simulink model "sampleModel1727_2_sub_sub_sub"  (R2023a)
settings: Solver=VariableStepAuto  StartTime=0.0  StopTime=10.0  RelTol=1e-3
libraries: simulink x4, hdlsllib x3
settings Model: Creator=user1  LastModifiedBy=user1

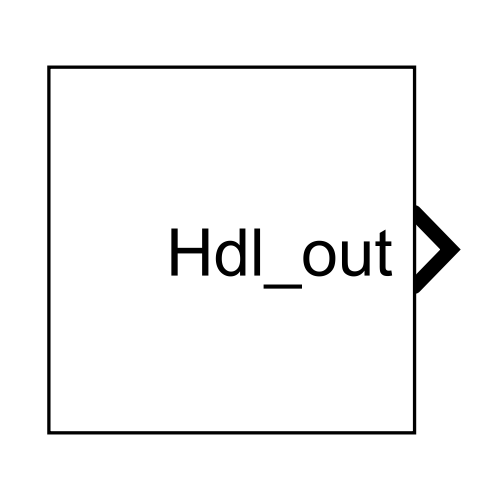
[thumbnail: Simulink's stored preview of the top-level diagram]
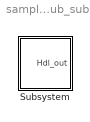
== system sampleModel1727_2_sub_sub_sub ==
  Subsystem : Subsystem

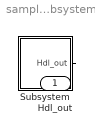
== system sampleModel1727_2_sub_sub_sub/Subsystem ==
  Subsystem : Subsystem
  Hdl_out : Outport  OutDataTypeStr=uint8
  wires:
  Subsystem/1(Hdl_out) -> Hdl_out/1

== system sampleModel1727_2_sub_sub_sub/Subsystem/Subsystem ==
  Subsystem : Subsystem
  Hdl_out : Outport  OutDataTypeStr=uint8

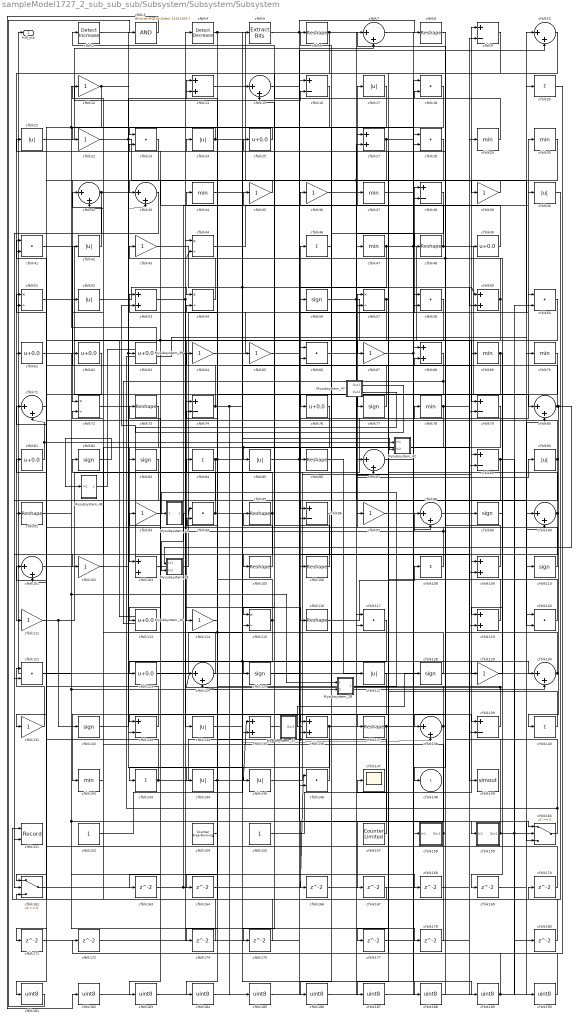
== system sampleModel1727_2_sub_sub_sub/Subsystem/Subsystem/Subsystem ==
  Mysubsystem_10 : Subsystem  TreatAsAtomicUnit=on  RTWFcnName=Mysubsystem_10
      settings: RTWFcnNameOpts=User specified  RTWFileNameOpts=Use function name
  Mysubsystem_11 : Subsystem  TreatAsAtomicUnit=on  RTWFcnName=Mysubsystem_11
      settings: RTWFcnNameOpts=User specified  RTWFileNameOpts=Use function name
  Mysubsystem_28 : Subsystem  TreatAsAtomicUnit=on  RTWFcnName=Mysubsystem_28
      settings: RTWFcnNameOpts=User specified  RTWFileNameOpts=Use function name
  Mysubsystem_31 : Subsystem  TreatAsAtomicUnit=on  RTWFcnName=Mysubsystem_31
      settings: RTWFcnNameOpts=User specified  RTWFileNameOpts=Use function name
  Mysubsystem_38 : Subsystem  TreatAsAtomicUnit=on  RTWFcnName=Mysubsystem_38
      settings: RTWFcnNameOpts=User specified  RTWFileNameOpts=Use function name
  Mysubsystem_39 : Subsystem  TreatAsAtomicUnit=on  RTWFcnName=Mysubsystem_39
      settings: RTWFcnNameOpts=User specified  RTWFileNameOpts=Use function name
  Mysubsystem_40 : Subsystem  TreatAsAtomicUnit=on  RTWFcnName=Mysubsystem_40
      settings: RTWFcnNameOpts=User specified  RTWFileNameOpts=Use function name
  Mysubsystem_42 : Subsystem  TreatAsAtomicUnit=on  RTWFcnName=Mysubsystem_42
      settings: RTWFcnNameOpts=User specified  RTWFileNameOpts=Use function name
  Mysubsystem_47 : Subsystem  TreatAsAtomicUnit=on  RTWFcnName=Mysubsystem_47
      settings: RTWFcnNameOpts=User specified  RTWFileNameOpts=Use function name
  cfblk{7,10,15,32..33,71,80,87,98,100..101,124,130,138} (14 alike) : Sum  Inputs=|++  OutDataTypeStr=uint8
  cfblk{12,22,35..36,39,43,64..65,67,93,97,102,111,114,129,131} (16 alike) : Gain  OutDataTypeStr=uint8
  cfblk{14,27,53,59,68,103,109,119,135..136} (10 alike) : Sum  OutDataTypeStr=uint8
  cfblk{6,8,48,73,86,91,95,105..106,116,137} (11 alike) : Reshape
  cfblk{20,46,84,108,140,143} (6 alike) : Sum  Inputs=+  OutDataTypeStr=uint8
  cfblk{56,77,82..83,99,110,125,128,132} (9 alike) : Signum
  cfblk{25,49,61..63,76,81,113,123} (9 alike) : Bias  Bias=0.0  SaturateOnIntegerOverflow=off
  cfblk{44,51,54,57,72,115} (6 alike) : Product  Inputs=*/  OutDataTypeStr=uint8  RndMeth=Zero  SaturateOnIntegerOverflow=on
  cfblk{18,23,28,41,58,60,66,94,117,120..121,146} (12 alike) : DotProduct  OutDataTypeStr=uint8
  cfblk{17,21,24,40,42,52,85,90,127,134,144..145} (12 alike) : Abs  OutDataTypeStr=uint8  SaturateOnIntegerOverflow=off
  cfblk{9,16,38,74,79,89,96,133,139} (9 alike) : Sum  Inputs=+-  OutDataTypeStr=uint8
  cfblk{29..30,34,37,47,69..70,78,142} (9 alike) : MinMax  OutDataTypeStr=uint8
  cfblk147 : Scope
  cfblk149 : ToWorkspace  VariableName=simout  SaveFormat=Timeseries  SampleTime=-1
  cfblk151 : Record  FileSettingsInternal="{\"entries\":[{\"content\":{\"excelSettings\":{\"content\":{},\"type\":\"Streamout.ExcelSettings\"}},\"type\":\"Streamout.FileSettingStorage\",\"uuid\":\"\"}],\"packageUris\":[\"http:\\/\\/schema.mathworks.com\\/mf0\\/streamout_blocks\\/R2020a\"],\"version\":\"1.0\"}"  Layout=[1 1]  SignalsInternal="{\"entries\":[{\"content\":{\"signals\":[{\"content\":{\"blockPath\":[],\"dimensions\":[1],\"domain\":\"\",\"lineColor\":\"#a2142f\",\"plots\":[1],\"port\":1,\"signalID\":37443,\"signalName\":\"cfblk158\"},\"type\":\"RecordBlkView.Signal\",\"uuid\":\"\"},{\"content\":{\"blockPath\":[],\"dimensions\":[1],\"domain\":\"\",\"lineColor\":\"#139fff\",\"plots\":[1],\"port\":2,\"signalID\":37446,\"signalName\":\"cfblk100\"},\"type\":\"RecordBlkView.Signal\",\"uuid\":\"\"}]},\"type\":\"RecordBlkView.InputSignals\",\"uuid\":\"\"}],\"packageUris\":[\"http:\\/\\/schema.mathworks.com\\/mf0\\/streamout_blocks\\/R2020a\"],\"version\":\"1.0\"}"  VisualizationBindings="{\"xyplotplugin\":{\"info\":[{\"series\":[{\"bindingParametersList\":[{\"parameter\":\"X-Axis\",\"signalID\":37443,\"signalName\":\"cfblk158\"},{\"parameter\":\"Y-Axis\",\"signalID\":37446,\"signalName\":\"cfblk100\"}],\"seriesID\":422}],\"subplotID\":1}]}}"  CompatibilityTag=XY  st=-1
  cfblk152 : Constant  OutDataTypeStr=uint8  SampleTime=-1
  cfblk154 : hdlsllib/Sources/Counter Free-Running  NumBits=16  tsamp=-1
  cfblk155 : Constant  OutDataTypeStr=uint8  SampleTime=-1
  cfblk157 : hdlsllib/Sources/Counter Limited  uplimit=7  tsamp=-1
  cfblk158 : Subsystem
      settings: LibrarySourceBlock=|
      | hdlsllib/Ports &
      | Subsystems/Subsystem
  cfblk159 : Subsystem
      settings: LibrarySourceBlock=|
      | hdlsllib/Ports &
      | Subsystems/Subsystem
  cfblk160 : Switch  OutDataTypeStr=uint8  SaturateOnIntegerOverflow=off  InputSameDT=off
  cfblk161 : Switch  OutDataTypeStr=uint8  SaturateOnIntegerOverflow=off  InputSameDT=off
  cfblk{163..164,166..172,174..175,177..178,180} (14 alike) : Delay  SampleTime=1
  cfblk{181..190} (10 alike) : DataTypeConversion  OutDataTypeStr=uint8  SaturateOnIntegerOverflow=off  RndMeth=Floor
  cfblk2 : simulink/Logic and Bit Operations/Detect Increase  vinit=0.0  OutDataTypeStr=uint8
      settings: LibrarySourceBlock=|
      | hdlsllib/Logic and Bit
      | Operations/Detect
      | Increase
  cfblk3 : simulink/Logic and Bit Operations/Bitwise Operator  logicop=AND  UseBitMask=on  BitMask=bin2dec('11011001')  BitMaskRealWorld=Stored Integer
      settings: LibrarySourceBlock=|
      | hdlsllib/Logic and Bit
      | Operations/Bitwise
      | Operator
  cfblk4 : simulink/Logic and Bit Operations/Detect Decrease  vinit=0.0  OutDataTypeStr=uint8
      settings: LibrarySourceBlock=|
      | hdlsllib/Logic and Bit
      | Operations/Detect
      | Decrease
  cfblk5 : simulink/Logic and Bit Operations/Extract Bits  bitsToExtract=Upper half  numBits=8  bitIdxRange=[0 7]  outScalingMode=Preserve fixed-point scaling
      settings: LibrarySourceBlock=|
      | hdlsllib/Logic and Bit
      | Operations/Extract Bits
  cfblk148 : Outport  OutDataTypeStr=uint8  VectorParamsAs1DForOutWhenUnconnected=off
  Hdl_out : Outport  Port=2  OutDataTypeStr=uint8
  wires:
  cfblk108/1 -> cfblk94/1, cfblk57/1
  cfblk161/1 -> cfblk146/1, cfblk35/1
  cfblk155/1 -> cfblk9/1
  cfblk52/1 -> cfblk54/1
  cfblk6/1 -> cfblk111/1, cfblk38/2, cfblk59/2
  cfblk73/1 -> cfblk103/1
  cfblk86/1 -> cfblk127/1
  cfblk69/1 -> cfblk119/1, cfblk148/1
  cfblk35/1 -> cfblk72/1
  cfblk49/1 -> cfblk17/1
  cfblk57/1 -> cfblk177/1, cfblk114/1
  cfblk120/1 -> cfblk109/1
  cfblk39/1 -> cfblk33/1
  cfblk42/1 -> cfblk32/1
  cfblk79/1 -> cfblk85/1, cfblk113/1
  cfblk10/1 -> cfblk137/1
  cfblk95/1 -> cfblk115/2, cfblk82/1
  cfblk41/1 -> cfblk77/1
  cfblk27/1 -> cfblk146/2, cfblk158/1(In1)
  cfblk74/1 -> cfblk42/1, cfblk185/1, cfblk159/1(In1)
  cfblk111/1 -> cfblk132/1, cfblk30/1
  cfblk29/1 -> cfblk2/1
  cfblk116/1 -> cfblk108/1
  cfblk103/1 -> cfblk60/1
  cfblk139/1 -> cfblk124/1, cfblk53/1
  cfblk4/1 -> cfblk124/2, cfblk39/1
  cfblk9/1 -> cfblk105/1
  cfblk33/1 -> cfblk61/1
  cfblk132/1 -> cfblk14/2, cfblk63/1
  cfblk71/1 -> cfblk161/1
  cfblk143/1 -> cfblk5/1, cfblk101/1
  cfblk146/1 -> cfblk74/2, cfblk46/1
  cfblk105/1 -> cfblk95/1
  cfblk77/1 -> cfblk6/1
  cfblk110/1 -> cfblk51/1
  cfblk51/1 -> cfblk67/1
  cfblk37/1 -> cfblk189/1
  cfblk64/1 -> cfblk20/1
  cfblk121/1 -> cfblk178/1, cfblk160/2, Mysubsystem_28/2(In2)
  cfblk154/1 -> cfblk34/1
  cfblk59/1 -> cfblk15/2, cfblk131/1
  cfblk159/1(Out1) -> cfblk97/1, cfblk180/1, cfblk80/2
  cfblk23/1 -> cfblk101/2
  cfblk78/1 -> cfblk102/1, cfblk149/1
  cfblk80/1 -> cfblk41/1, cfblk140/1, Mysubsystem_38/1(In1)
  cfblk68/1 -> cfblk144/1, Mysubsystem_10/2(In2)
  cfblk14/1 -> cfblk70/1
  cfblk43/1 -> cfblk98/2
  cfblk28/1 -> cfblk123/1
  cfblk158/1(Out1) -> cfblk52/1, cfblk151/1
  cfblk38/1 -> cfblk76/1
  cfblk60/1 -> cfblk133/1, Mysubsystem_10/1(In1)
  cfblk56/1 -> cfblk80/1, cfblk79/1
  cfblk48/1 -> cfblk23/2, cfblk120/1
  cfblk123/1 -> cfblk15/1
  cfblk152/1 -> cfblk65/1
  cfblk144/1 -> cfblk64/1, cfblk135/1
  cfblk97/1 -> cfblk68/1
  cfblk142/1 -> cfblk32/2
  cfblk157/1 -> cfblk84/1
  cfblk113/1 -> cfblk93/1
  cfblk12/1 -> cfblk145/1, cfblk91/1
  cfblk100/1 -> cfblk56/1, cfblk151/2
  cfblk46/1 -> cfblk86/1
  cfblk133/1 -> cfblk81/1
  cfblk160/1 -> cfblk21/1, Mysubsystem_39/2(In2)
  cfblk125/1 -> cfblk89/1
  cfblk63/1 -> cfblk38/1
  cfblk47/1 -> cfblk96/2, cfblk40/1, cfblk99/1
  cfblk34/1 -> cfblk89/2
  cfblk84/1 -> cfblk133/2, cfblk188/1, cfblk184/1
  cfblk115/1 -> cfblk94/2, cfblk174/1, cfblk135/2
  cfblk135/1 -> cfblk47/1
  cfblk66/1 -> cfblk100/2
  cfblk119/1 -> cfblk27/1
  cfblk32/1 -> cfblk121/2, cfblk130/1
  cfblk145/1 -> cfblk57/2
  cfblk101/1 -> cfblk160/3, Mysubsystem_28/1(In1)
  cfblk87/1 -> cfblk58/1
  cfblk128/1 -> cfblk24/1, cfblk73/1
  cfblk138/1 -> cfblk166/1, cfblk36/1
  cfblk90/1 -> cfblk41/2, cfblk143/1
  cfblk83/1 -> cfblk161/2
  cfblk94/1 -> cfblk62/1, Mysubsystem_42/2(In2)
  cfblk7/1 -> cfblk58/2
  cfblk54/1 -> cfblk43/1
  cfblk93/1 -> cfblk134/1
  cfblk76/1 -> cfblk115/1
  cfblk15/1 -> cfblk160/1
  cfblk114/1 -> cfblk14/1
  cfblk131/1 -> cfblk121/1
  cfblk44/1 -> cfblk10/1
  cfblk109/1 -> cfblk44/2, cfblk7/1
  cfblk22/1 -> cfblk87/2, cfblk33/2
  cfblk21/1 -> cfblk7/2
  cfblk2/1 -> cfblk125/1
  cfblk134/1 -> cfblk69/1
  cfblk129/1 -> cfblk49/1
  cfblk67/1 -> cfblk129/1, cfblk28/1
  cfblk85/1 -> cfblk139/1, cfblk78/1
  cfblk130/1 -> Hdl_out/1, cfblk68/2
  cfblk102/1 -> cfblk83/1
  cfblk25/1 -> cfblk22/1
  cfblk136/1 -> cfblk163/1, cfblk90/1
  cfblk106/1 -> cfblk25/1
  cfblk89/1 -> cfblk190/1, cfblk136/2
  cfblk24/1 -> cfblk23/1, cfblk138/2, cfblk59/1
  cfblk137/1 -> cfblk167/1, cfblk139/2
  cfblk91/1 -> cfblk130/2
  cfblk5/1 -> cfblk109/2, cfblk8/1
  cfblk30/1 -> cfblk96/1
  cfblk53/1 -> cfblk116/1, cfblk4/1
  cfblk72/1 -> cfblk136/1
  cfblk16/1 -> cfblk66/2
  cfblk127/1 -> cfblk142/1
  cfblk8/1 -> cfblk138/1
  cfblk81/1 -> cfblk71/2, Mysubsystem_42/1(In1)
  cfblk98/1 -> cfblk29/1
  cfblk140/1 -> cfblk87/1
  cfblk65/1 -> cfblk10/2
  cfblk36/1 -> cfblk48/1
  cfblk124/1 -> cfblk12/1
  cfblk163/1 -> cfblk66/1
  cfblk58/1 -> cfblk164/1
  cfblk164/1 -> cfblk27/2
  cfblk166/1 -> cfblk79/2
  cfblk167/1 -> cfblk161/3
  cfblk61/1 -> cfblk168/1
  cfblk168/1 -> cfblk98/1
  cfblk99/1 -> cfblk169/1
  cfblk169/1 -> cfblk100/1
  cfblk40/1 -> cfblk170/1
  cfblk170/1 -> cfblk71/1
  cfblk96/1 -> cfblk171/1
  cfblk171/1 -> cfblk44/1
  cfblk20/1 -> cfblk172/1
  cfblk172/1 -> cfblk16/1
  cfblk174/1 -> cfblk72/2
  cfblk17/1 -> cfblk175/1
  cfblk175/1 -> cfblk51/2
  cfblk177/1 -> cfblk119/2
  cfblk178/1 -> cfblk54/2
  cfblk180/1 -> cfblk74/1
  cfblk62/1 -> cfblk181/1
  cfblk181/1 -> cfblk3/1
  cfblk3/1 -> cfblk182/1
  cfblk182/1 -> cfblk110/1
  cfblk117/1 -> cfblk183/1
  cfblk183/1 -> cfblk106/1
  cfblk184/1 -> cfblk117/1
  cfblk185/1 -> cfblk117/2
  cfblk18/1 -> cfblk186/1
  cfblk186/1 -> cfblk9/2
  cfblk70/1 -> cfblk187/1
  cfblk187/1 -> cfblk18/1
  cfblk188/1 -> cfblk18/2
  cfblk189/1 -> cfblk60/2, cfblk147/1
  cfblk190/1 -> cfblk37/1
  Mysubsystem_28/1(Out1) -> Mysubsystem_11/1(In1)
  Mysubsystem_31/1(Out1) -> cfblk128/1
  Mysubsystem_11/1(Out1) -> Mysubsystem_38/2(In2)
  Mysubsystem_39/1(Out1) -> cfblk28/2, cfblk16/2
  Mysubsystem_39/2(Out2) -> cfblk120/2
  cfblk82/1 -> Mysubsystem_40/1(In1)
  Mysubsystem_40/1(y) -> Mysubsystem_39/1(In1)
  Mysubsystem_47/1(Out1) -> cfblk53/2
  Mysubsystem_47/2(Out2) -> cfblk103/2

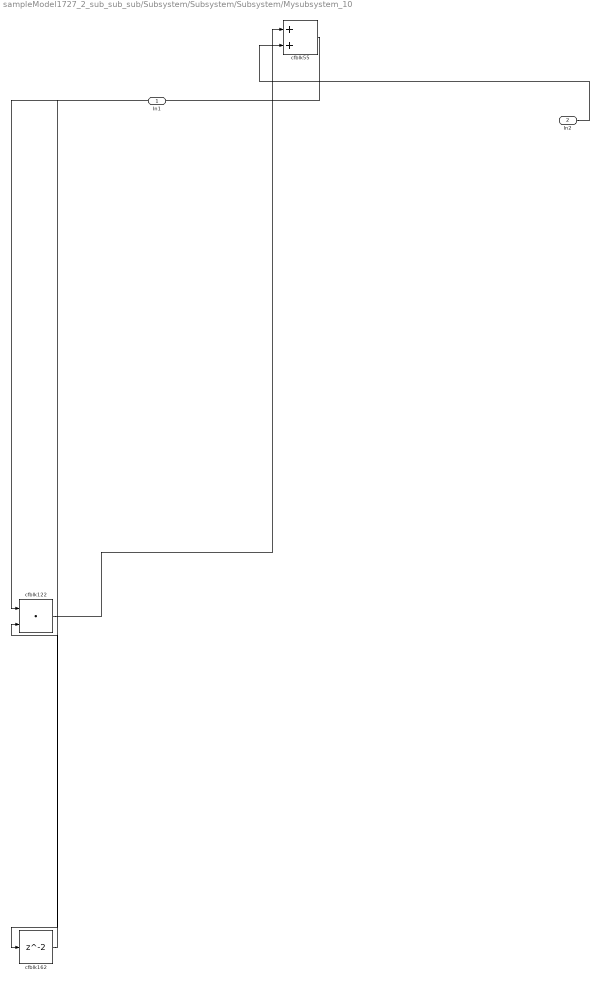
== system sampleModel1727_2_sub_sub_sub/Subsystem/Subsystem/Subsystem/Mysubsystem_10 ==
  In1 : Inport
  In2 : Inport  Port=2
  cfblk122 : DotProduct  OutDataTypeStr=Inherit: Inherit via internal rule
  cfblk162 : Delay  SampleTime=1
  cfblk55 : Sum
  wires:
  In2/1 -> cfblk55/2
  In1/1 -> cfblk122/1
  cfblk162/1 -> cfblk122/2
  cfblk122/1 -> cfblk55/1
  cfblk55/1 -> cfblk162/1

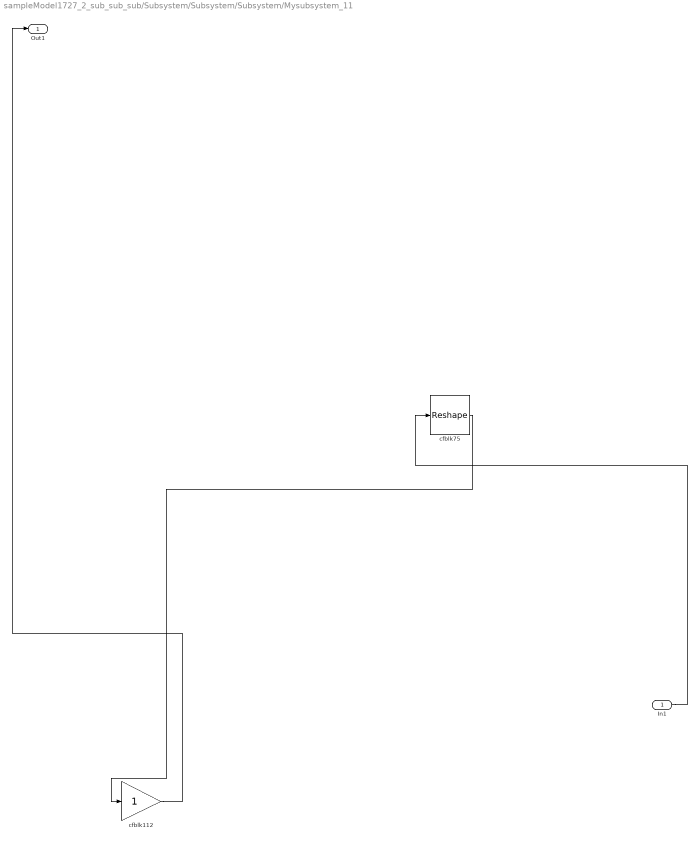
== system sampleModel1727_2_sub_sub_sub/Subsystem/Subsystem/Subsystem/Mysubsystem_11 ==
  In1 : Inport
  cfblk112 : Gain
  cfblk75 : Reshape
  Out1 : Outport
  wires:
  In1/1 -> cfblk75/1
  cfblk112/1 -> Out1/1
  cfblk75/1 -> cfblk112/1

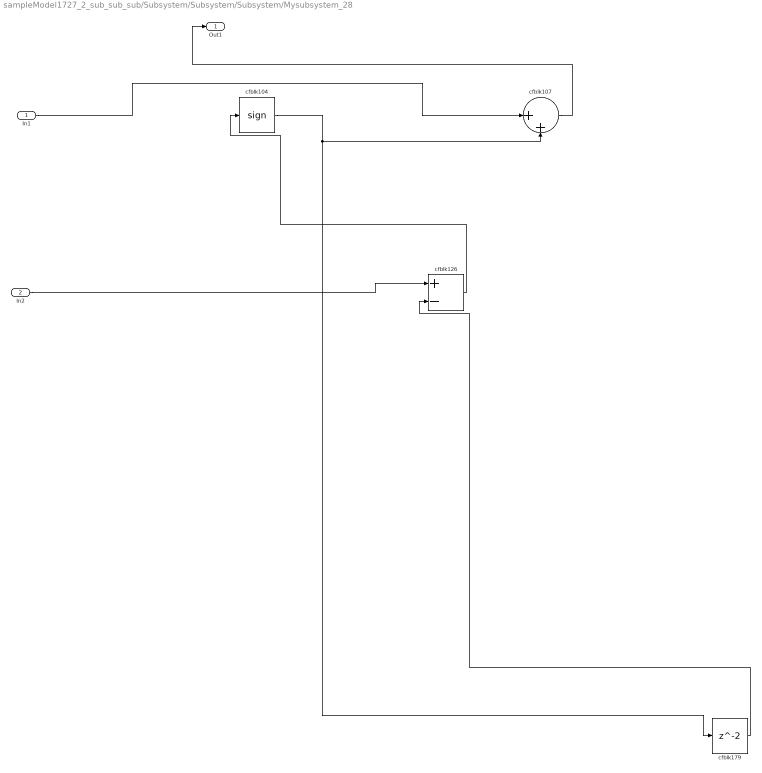
== system sampleModel1727_2_sub_sub_sub/Subsystem/Subsystem/Subsystem/Mysubsystem_28 ==
  In1 : Inport
  In2 : Inport  Port=2
  cfblk104 : Signum
  cfblk107 : Sum  Inputs=|++
  cfblk126 : Sum  Inputs=+-
  cfblk179 : Delay  SampleTime=1
  Out1 : Outport
  wires:
  cfblk104/1 -> cfblk179/1, cfblk107/2
  In2/1 -> cfblk126/1
  In1/1 -> cfblk107/1
  cfblk107/1 -> Out1/1
  cfblk126/1 -> cfblk104/1
  cfblk179/1 -> cfblk126/2

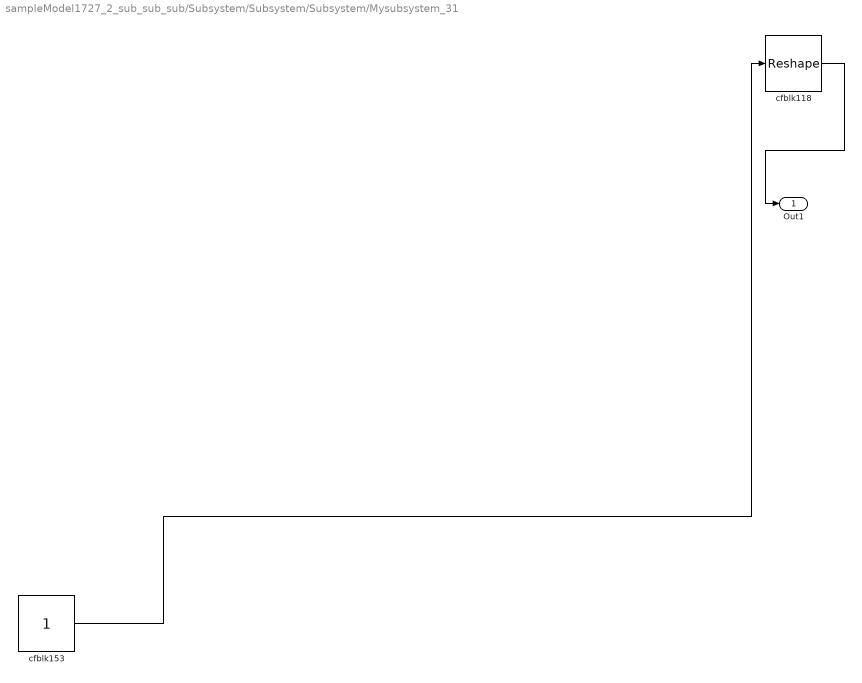
== system sampleModel1727_2_sub_sub_sub/Subsystem/Subsystem/Subsystem/Mysubsystem_31 ==
  cfblk118 : Reshape
  cfblk153 : Constant  SampleTime=-1
  Out1 : Outport
  wires:
  cfblk118/1 -> Out1/1
  cfblk153/1 -> cfblk118/1

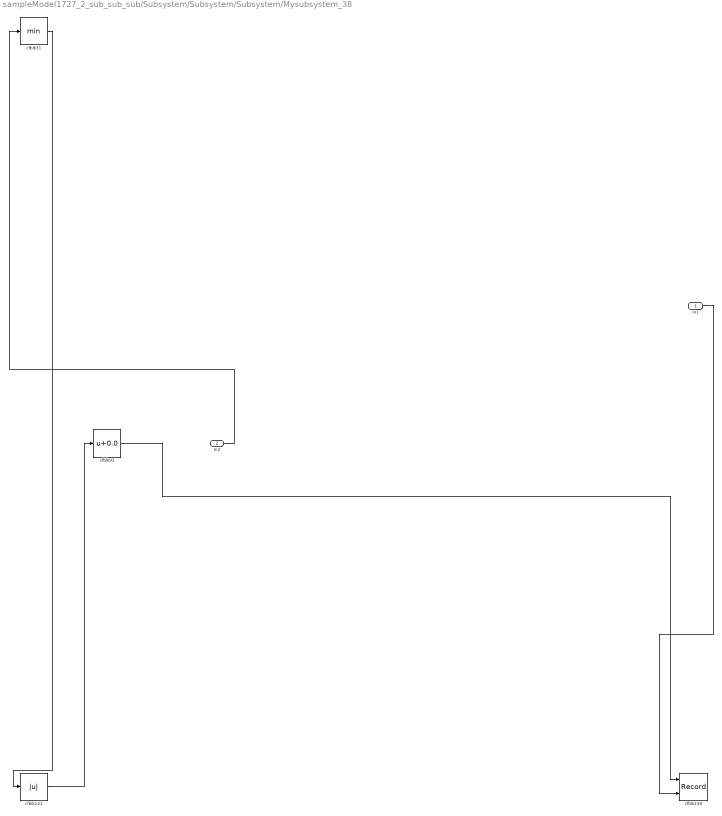
== system sampleModel1727_2_sub_sub_sub/Subsystem/Subsystem/Subsystem/Mysubsystem_38 ==
  In1 : Inport
  In2 : Inport  Port=2
  cfblk141 : Abs  SaturateOnIntegerOverflow=off
  cfblk150 : Record  FileSettingsInternal="{\"entries\":[{\"content\":{\"excelSettings\":{\"content\":{},\"type\":\"Streamout.ExcelSettings\"}},\"type\":\"Streamout.FileSettingStorage\",\"uuid\":\"\"}],\"packageUris\":[\"http:\\/\\/schema.mathworks.com\\/mf0\\/streamout_blocks\\/R2020a\"],\"version\":\"1.0\"}"  Layout=[1 1]  SignalsInternal="{\"entries\":[{\"content\":{},\"type\":\"RecordBlkView.InputSignals\",\"uuid\":\"\"}],\"packageUris\":[\"http:\\/\\/schema.mathworks.com\\/mf0\\/streamout_blocks\\/R2020a\"],\"version\":\"1.0\"}"  VisualizationBindings="{\"xyplotplugin\":{\"info\":[{\"series\":[],\"subplotID\":1}]}}"  CompatibilityTag=XY  st=-1
  cfblk31 : MinMax
  cfblk92 : Bias  Bias=0.0  SaturateOnIntegerOverflow=off
  wires:
  In1/1 -> cfblk150/2
  In2/1 -> cfblk31/1
  cfblk31/1 -> cfblk141/1
  cfblk92/1 -> cfblk150/1
  cfblk141/1 -> cfblk92/1

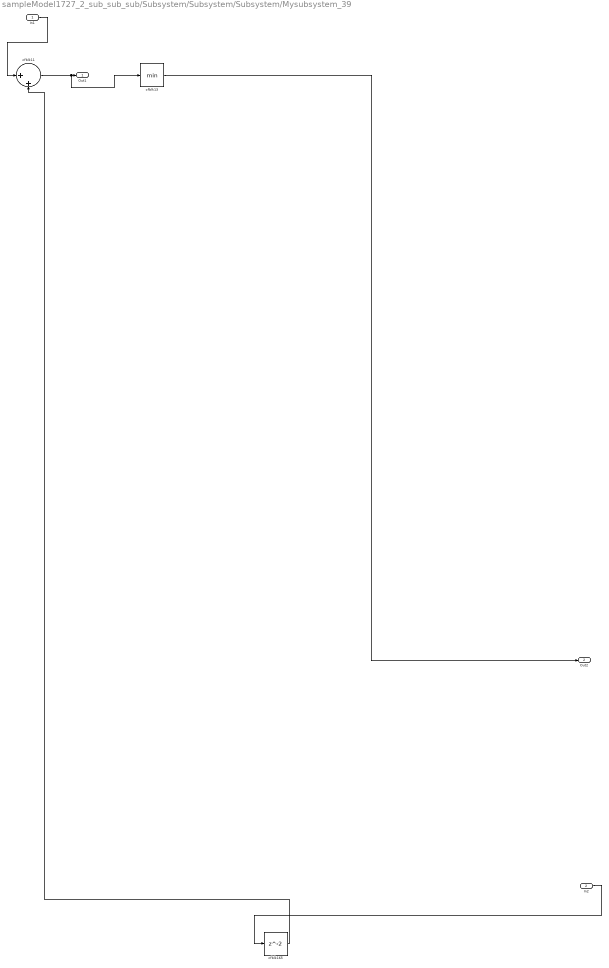
== system sampleModel1727_2_sub_sub_sub/Subsystem/Subsystem/Subsystem/Mysubsystem_39 ==
  In1 : Inport
  In2 : Inport  Port=2
  cfblk11 : Sum  Inputs=|++
  cfblk13 : MinMax
  cfblk165 : Delay  SampleTime=1
  Out1 : Outport
  Out2 : Outport  Port=2
  wires:
  cfblk11/1 -> Out1/1, cfblk13/1
  In2/1 -> cfblk165/1
  cfblk13/1 -> Out2/1
  cfblk165/1 -> cfblk11/2
  In1/1 -> cfblk11/1

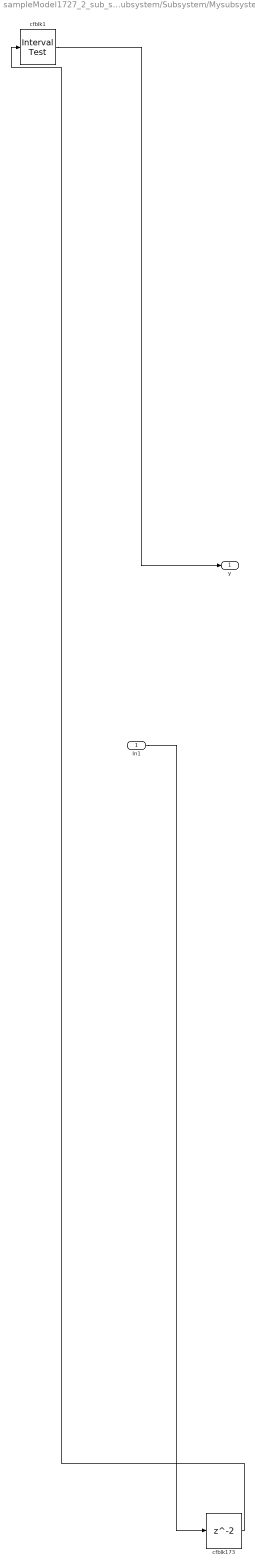
== system sampleModel1727_2_sub_sub_sub/Subsystem/Subsystem/Subsystem/Mysubsystem_40 ==
  In1 : Inport
  cfblk1 : hdlsllib/Logic and Bit Operations/Interval Test  IntervalClosedRight=on  uplimit=0.5  IntervalClosedLeft=on  lowlimit=-0.5  OutDataTypeStr=boolean
  cfblk173 : Delay  SampleTime=1
  y : Outport
  wires:
  In1/1 -> cfblk173/1
  cfblk1/1 -> y/1
  cfblk173/1 -> cfblk1/1

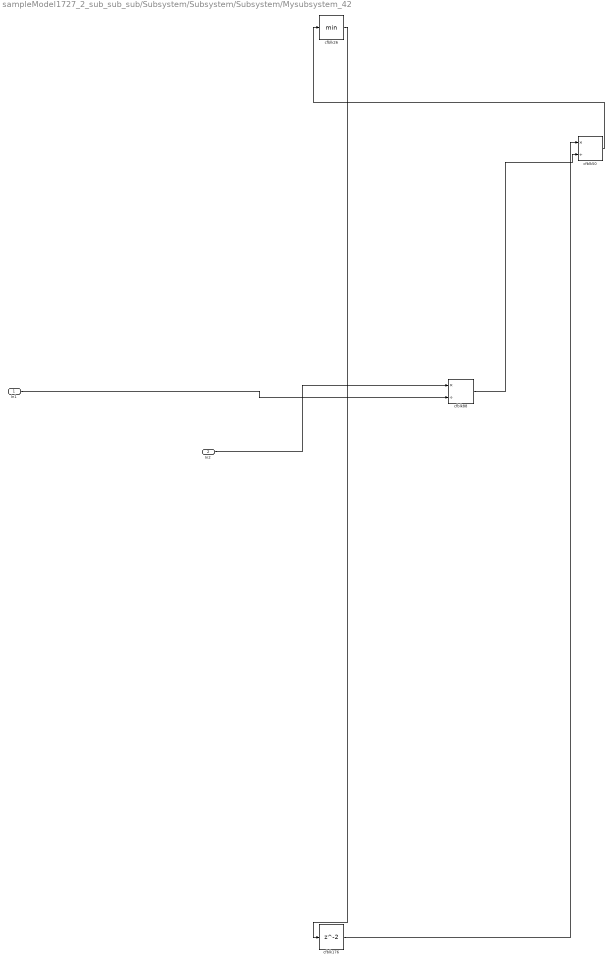
== system sampleModel1727_2_sub_sub_sub/Subsystem/Subsystem/Subsystem/Mysubsystem_42 ==
  In1 : Inport
  In2 : Inport  Port=2
  cfblk176 : Delay  SampleTime=1
  cfblk26 : MinMax
  cfblk50 : Product  Inputs=*/  RndMeth=Zero  SaturateOnIntegerOverflow=on
  cfblk88 : Product  Inputs=*/  RndMeth=Zero  SaturateOnIntegerOverflow=on
  wires:
  In1/1 -> cfblk88/2
  cfblk50/1 -> cfblk26/1
  cfblk88/1 -> cfblk50/2
  In2/1 -> cfblk88/1
  cfblk26/1 -> cfblk176/1
  cfblk176/1 -> cfblk50/1

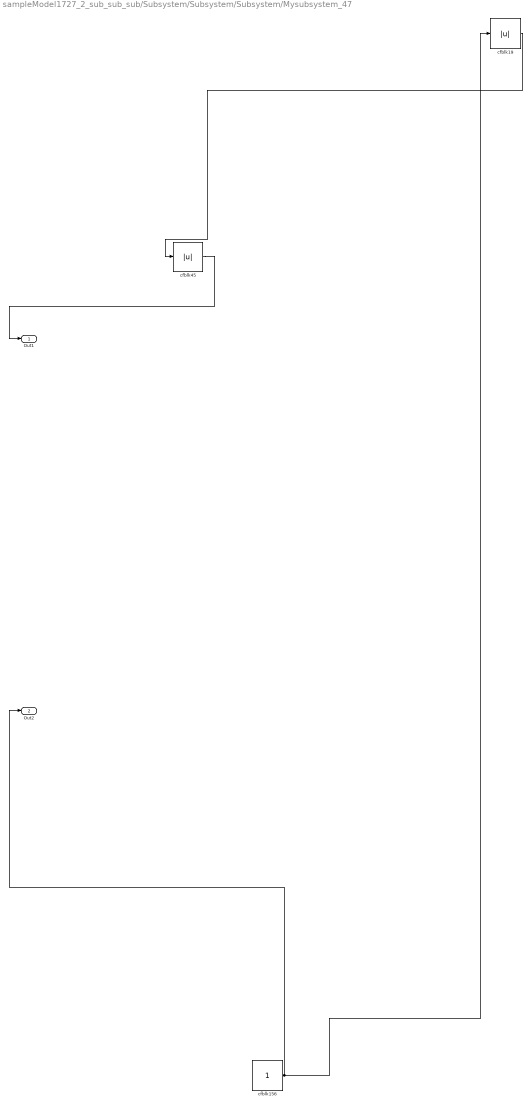
== system sampleModel1727_2_sub_sub_sub/Subsystem/Subsystem/Subsystem/Mysubsystem_47 ==
  cfblk156 : Constant  SampleTime=-1
  cfblk19 : Abs  SaturateOnIntegerOverflow=off
  cfblk45 : Abs  SaturateOnIntegerOverflow=off
  Out1 : Outport
  Out2 : Outport  Port=2
  wires:
  cfblk156/1 -> cfblk19/1, Out2/1
  cfblk19/1 -> cfblk45/1
  cfblk45/1 -> Out1/1

== system sampleModel1727_2_sub_sub_sub/Subsystem/Subsystem/Subsystem/cfblk158 ==
  In1 : Inport
  Out1 : Outport
  wires:
  In1/1 -> Out1/1

== system sampleModel1727_2_sub_sub_sub/Subsystem/Subsystem/Subsystem/cfblk159 ==
  In1 : Inport
  Out1 : Outport
  wires:
  In1/1 -> Out1/1
